simulink model "AMK_Derating"  (R2025b)
settings: Solver=VariableStepAuto  StartTime=0.0  StopTime=30  RelTol=1e-3  AbsTol=1e-3
libraries: simulink x1
settings Model: Creator=Utente  LastModifiedBy=Utente
settings SolverCC: AutoScaleAbsTol=off  AlgebraicLoopSolver=TrustRegion  MaxZcPerStep=1.0
settings DebuggingCC: UnconnectedInputMsg=warning  UnconnectedOutputMsg=warning  UnconnectedLineMsg=warning  SymbolicDimsDataTypeCodeGenerationDiagnostic=none
settings ModelReferenceCC: EnableRefExpFcnMdlSchedulingChecks=on
settings SFSimCC: CustomCodeUndefinedFunction=UseInterfaceOnly
settings RTWCC: GPUComputeCapability=3.5  DLArmComputeVersion=19.05
settings SimscapeCC: SimscapeLogType=all  SimscapeLogSimulationStatistics=on  SimscapeLogDataHistory=10000.0

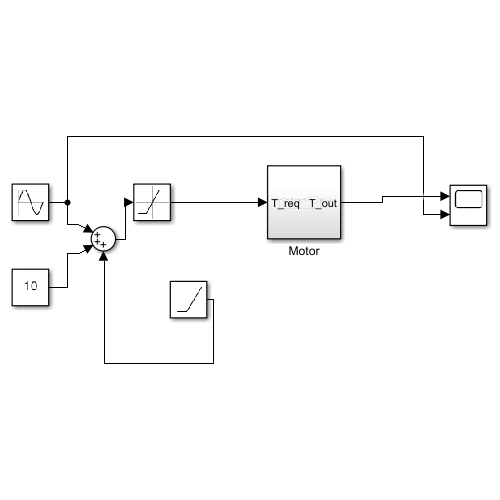
[thumbnail: Simulink's stored preview of the top-level diagram]
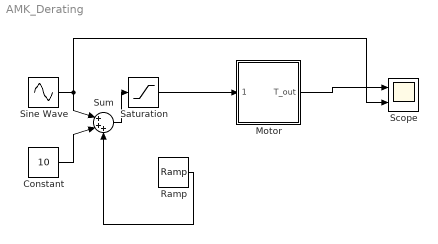
== system AMK_Derating ==
  Constant : Constant  Value=10
  Motor : Subsystem
  Ramp : simulink/Sources/Ramp  slope=10  start=4  InitialOutput=0
  Saturation : Saturate  UpperLimit=21  LowerLimit=0
  Scope : Scope  NumInputPorts=2
      settings: ActiveDisplayYMinimum=-7.9861259828821325  ActiveDisplayYMaximum=55.822345460076043
  Sine Wave : Sin  Amplitude=40  Frequency=0.1  SampleTime=0
  Sum : Sum  Inputs=|+++
  wires:
  Saturation/1 -> Motor/1(T_req)
  Motor/1(T_out) -> Scope/1
  Sine Wave/1 -> Sum/1, Scope/2
  Constant/1 -> Sum/2
  Sum/1 -> Saturation/1
  Ramp/1 -> Sum/3

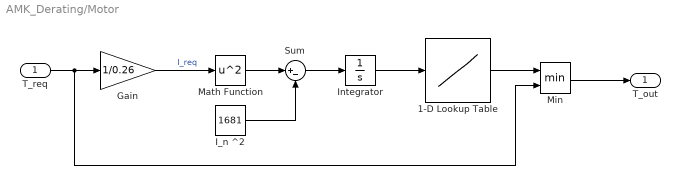
== system AMK_Derating/Motor ==
  T_req : Inport
  1-D Lookup Table : Lookup_n-D  NumberOfTableDimensions=1  BreakpointsForDimension1=[0, 9268, 11586.6]  Table=[21, 21, 9.8]  InternalRulePriority=Speed  RndMeth=Simplest
  Gain : Gain  Gain=1/0.26
  I_n ^2 : Constant  Value=1681
  Integrator : Integrator  LimitOutput=on  UpperSaturationLimit=11586.6  LowerSaturationLimit=0
  Math Function : Math  Operator=square
  Min : MinMax  Inputs=2
  Sum : Sum  Inputs=|+-
  T_out : Outport
  wires:
  Sum/1 -> Integrator/1
  T_req/1 -> Min/2, Gain/1
  I_n ^2/1 -> Sum/2
  Gain/1 -> Math Function/1  "I_req"
  Math Function/1 -> Sum/1
  Integrator/1 -> 1-D Lookup Table/1
  1-D Lookup Table/1 -> Min/1
  Min/1 -> T_out/1
